simulink model "ese1_sistemaLineare"  (Simulink 7.5)
settings: Solver=ode45  StartTime=0.0  StopTime=20  RelTol=1e-3
values from neighbouring files (symbols this model uses):
  A = [0 1;-k/m -b/m]    [EsercizioMassaMollaSmorzatore.m]    (also in serbatoi.m = [-k1/S1 0; k1/S2 -k2/S2 ])
  B = [0;1/m]    [EsercizioMassaMollaSmorzatore.m]    (also in serbatoi.m = [1/S1 0]')
  C = [1 0]    [EsercizioMassaMollaSmorzatore.m]    (also in serbatoi.m = [0 k2])
  D = 0    [EsercizioMassaMollaSmorzatore.m]    (also in serbatoi.m)
  ueq = 2    [EsercizioMassaMollaSmorzatore.m]    (also in serbatoi.m = 1)
  x0 = [0 0]'    [EsercizioMassaMollaSmorzatore.m]    (also in serbatoi.m = [1 1]')
libraries: simulink x1
settings Model: Creator=76936  LastModifiedBy=76936

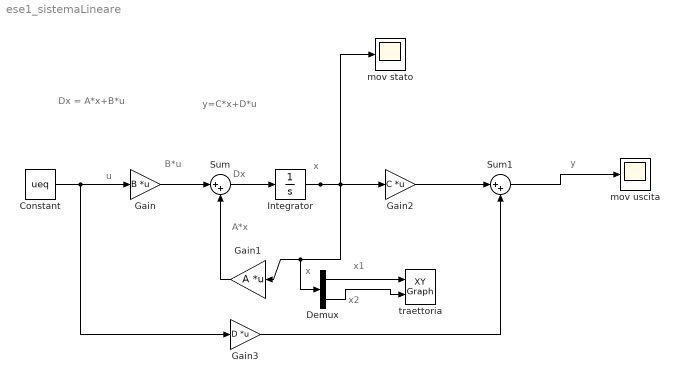
== system ese1_sistemaLineare ==
  note: Dx = A*x+B*u
  note: y=C*x+D*u
  note: A*x
  note: B*u
  note: u
  note: Dx
  note: x
  note: x
  note: x1
  note: x2
  note: y
  Constant : Constant  Value=ueq  OutDataType=fixdt(1, 16)  OutScaling=2^0
  Demux : Demux  Outputs=2
  Gain : Gain  Gain=B  Multiplication=Matrix(K*u)  ParameterDataType=fixdt(1, 16)  ParameterScaling=2^0  OutDataType=fixdt(1, 16)  OutScaling=2^0
  Gain1 : Gain  Gain=A  Multiplication=Matrix(K*u)  ParameterDataType=fixdt(1, 16)  ParameterScaling=2^0  OutDataType=fixdt(1, 16)  OutScaling=2^0
  Gain2 : Gain  Gain=C  Multiplication=Matrix(K*u)  ParameterDataType=fixdt(1, 16)  ParameterScaling=2^0  OutDataType=fixdt(1, 16)  OutScaling=2^0
  Gain3 : Gain  Gain=D  Multiplication=Matrix(K*u)  ParameterDataType=fixdt(1, 16)  ParameterScaling=2^0  OutDataType=fixdt(1, 16)  OutScaling=2^0
  Integrator : Integrator  InitialCondition=x0
  Sum : Sum  Inputs=|++  OutDataType=fixdt(1, 16)  OutScaling=2^0
  Sum1 : Sum  Inputs=|++  OutDataType=fixdt(1, 16)  OutScaling=2^0
  mov stato : Scope
  mov uscita : Scope
  traettoria : simulink/Sinks/XY Graph  SystemSampleTime=-1  xmin=0  xmax=2  ymin=0  ymax=2  st=-1
  wires:
  Gain/1 -> Sum/1
  Gain1/1 -> Sum/2
  Sum/1 -> Integrator/1
  Gain3/1 -> Sum1/2
  Constant/1 -> Gain/1, Gain3/1
  Integrator/1 -> mov stato/1, Gain1/1, Demux/1, Gain2/1
  Gain2/1 -> Sum1/1
  Sum1/1 -> mov uscita/1
  Demux/1 -> traettoria/1
  Demux/2 -> traettoria/2
